simulink model "tensegrity_joint_universal"  (R2022b)
settings: Solver=VariableStepAuto  StartTime=0.0  StopTime=t_end  RelTol=1e-3
InitFcn:
  | %parameters_tensegrity_joint;
  | %l0_all=cables_l0(fix, fiz, w, h, b);
  | %predpeti=0.95;
values from neighbouring files (symbols this model uses):
  Fx_load = joint_stiffness(1, 12)    [plot_graphs_revolute.m]    (also in tensegrity_joint_revolute_stiffness.m = 10)
  Fy_load = joint_stiffness(1, 13)    [plot_graphs_revolute.m]    (also in tensegrity_joint_revolute_stiffness.m = 0)
  Fz_load = joint_stiffness(1, 14)    [plot_graphs_revolute.m]    (also in tensegrity_joint_revolute_stiffness.m = 0)
  l0_all = [l01, l02, l03, l04, l05, l06, l07, l08]    [tensegrity_universal_joint_plot.m]
  Mx_load = joint_stiffness(1, 15)    [plot_graphs_revolute.m]    (also in tensegrity_joint_revolute_stiffness.m = 0)
  My_load = joint_stiffness(1, 16)    [plot_graphs_revolute.m]    (also in tensegrity_joint_revolute_stiffness.m = 0)
  Mz_load = joint_stiffness(1, 17)    [plot_graphs_revolute.m]    (also in tensegrity_joint_revolute_stiffness.m = 0)
  predpeti_all = ll./l0_all    [tensegrity_joint_revolute_stiffness.m]
  t_measure = 0.25    [tensegrity_joint_revolute_stiffness.m]
undefined symbols (not defined in the file or in its folder): a, b, b_all, h, k_all, w
libraries: nesl_utility x35, sm_lib x33
(part 2 of 2)

== system tensegrity_joint_universal/Subsystem/internal cable force_3/cable force ==
  i : Inport
  PS-Simulink Converter1 : nesl_utility/PS-Simulink Converter  PhysicalDomain=network_engine_domain  SubClassName=ps_output  LeftPortType=input  RightPortType=output  PseudoPeriodic=off  Frequencies=[]  VectorFormat=1-D array  Unit=inherit  AffineConversion=off
  PS-Simulink Converter2 : nesl_utility/PS-Simulink Converter  PhysicalDomain=network_engine_domain  SubClassName=ps_output  LeftPortType=input  RightPortType=output  PseudoPeriodic=off  Frequencies=[]  VectorFormat=1-D array  Unit=inherit  AffineConversion=off
  Transform Sensor : sm_lib/Frames and Transforms/Transform Sensor  MeasurementFrame=World  SenseAngle=off  SenseAxis=off  SenseQ=off  SenseR=off  SenseRotationSequence=off  RotationSequence=XYX  SenseOmegaX=off  SenseOmegaY=off  SenseOmegaZ=off  SenseQDot=off  SenseRDot=off  SenseAlphaX=off  SenseAlphaY=off  SenseAlphaZ=off  SenseQDDot=off  SenseRDDot=off  SenseX=off  SenseY=off  SenseZ=off  SenseRad=off  SenseAzim=off  SenseDist=on  SenseInc=off  SenseXDot=off  SenseYDot=off  SenseZDot=off  SenseRadDot=off  SenseAzimDot=off  SenseDistDot=on  SenseIncDot=off  SenseXDDot=off  SenseYDDot=off  SenseZDDot=off  SenseRadDDot=off  SenseAzimDDot=off  SenseDistDDot=off  SenseIncDDot=off
  cable force computation : MATLAB Function  TreatAsAtomicUnit=on
  parameter selection : Subsystem
  TO : PMIOPort  Side=Right
  FROM : PMIOPort  Port=2  Side=Right
  Fc : Outport
  wires:
  cable force computation/1(Fc) -> Fc/1
  parameter selection/2(b) -> cable force computation/2(b)
  parameter selection/1(k) -> cable force computation/1(k)
  PS-Simulink Converter1/1 -> cable force computation/4(l)
  PS-Simulink Converter2/1 -> cable force computation/5(v)
  i/1 -> parameter selection/1(i)
  parameter selection/4(l0_p) -> cable force computation/3(l0)
  connections:
  Transform Sensor/RConn3 -- PS-Simulink Converter2/LConn1
  Transform Sensor/RConn2 -- PS-Simulink Converter1/LConn1
  Transform Sensor/RConn1 -- TO/RConn1
  Transform Sensor/LConn1 -- FROM/RConn1

== system tensegrity_joint_universal/Subsystem/internal cable force_4/cable force ==
  i : Inport
  PS-Simulink Converter1 : nesl_utility/PS-Simulink Converter  PhysicalDomain=network_engine_domain  SubClassName=ps_output  LeftPortType=input  RightPortType=output  PseudoPeriodic=off  Frequencies=[]  VectorFormat=1-D array  Unit=inherit  AffineConversion=off
  PS-Simulink Converter2 : nesl_utility/PS-Simulink Converter  PhysicalDomain=network_engine_domain  SubClassName=ps_output  LeftPortType=input  RightPortType=output  PseudoPeriodic=off  Frequencies=[]  VectorFormat=1-D array  Unit=inherit  AffineConversion=off
  Transform Sensor : sm_lib/Frames and Transforms/Transform Sensor  MeasurementFrame=World  SenseAngle=off  SenseAxis=off  SenseQ=off  SenseR=off  SenseRotationSequence=off  RotationSequence=XYX  SenseOmegaX=off  SenseOmegaY=off  SenseOmegaZ=off  SenseQDot=off  SenseRDot=off  SenseAlphaX=off  SenseAlphaY=off  SenseAlphaZ=off  SenseQDDot=off  SenseRDDot=off  SenseX=off  SenseY=off  SenseZ=off  SenseRad=off  SenseAzim=off  SenseDist=on  SenseInc=off  SenseXDot=off  SenseYDot=off  SenseZDot=off  SenseRadDot=off  SenseAzimDot=off  SenseDistDot=on  SenseIncDot=off  SenseXDDot=off  SenseYDDot=off  SenseZDDot=off  SenseRadDDot=off  SenseAzimDDot=off  SenseDistDDot=off  SenseIncDDot=off
  cable force computation : MATLAB Function  TreatAsAtomicUnit=on
  parameter selection : Subsystem
  TO : PMIOPort  Side=Right
  FROM : PMIOPort  Port=2  Side=Right
  Fc : Outport
  wires:
  cable force computation/1(Fc) -> Fc/1
  parameter selection/2(b) -> cable force computation/2(b)
  parameter selection/1(k) -> cable force computation/1(k)
  PS-Simulink Converter1/1 -> cable force computation/4(l)
  PS-Simulink Converter2/1 -> cable force computation/5(v)
  i/1 -> parameter selection/1(i)
  parameter selection/4(l0_p) -> cable force computation/3(l0)
  connections:
  Transform Sensor/RConn3 -- PS-Simulink Converter2/LConn1
  Transform Sensor/RConn2 -- PS-Simulink Converter1/LConn1
  Transform Sensor/RConn1 -- TO/RConn1
  Transform Sensor/LConn1 -- FROM/RConn1

== system tensegrity_joint_universal/Subsystem/internal cable force_5/cable force ==
  i : Inport
  PS-Simulink Converter1 : nesl_utility/PS-Simulink Converter  PhysicalDomain=network_engine_domain  SubClassName=ps_output  LeftPortType=input  RightPortType=output  PseudoPeriodic=off  Frequencies=[]  VectorFormat=1-D array  Unit=inherit  AffineConversion=off
  PS-Simulink Converter2 : nesl_utility/PS-Simulink Converter  PhysicalDomain=network_engine_domain  SubClassName=ps_output  LeftPortType=input  RightPortType=output  PseudoPeriodic=off  Frequencies=[]  VectorFormat=1-D array  Unit=inherit  AffineConversion=off
  Transform Sensor : sm_lib/Frames and Transforms/Transform Sensor  MeasurementFrame=World  SenseAngle=off  SenseAxis=off  SenseQ=off  SenseR=off  SenseRotationSequence=off  RotationSequence=XYX  SenseOmegaX=off  SenseOmegaY=off  SenseOmegaZ=off  SenseQDot=off  SenseRDot=off  SenseAlphaX=off  SenseAlphaY=off  SenseAlphaZ=off  SenseQDDot=off  SenseRDDot=off  SenseX=off  SenseY=off  SenseZ=off  SenseRad=off  SenseAzim=off  SenseDist=on  SenseInc=off  SenseXDot=off  SenseYDot=off  SenseZDot=off  SenseRadDot=off  SenseAzimDot=off  SenseDistDot=on  SenseIncDot=off  SenseXDDot=off  SenseYDDot=off  SenseZDDot=off  SenseRadDDot=off  SenseAzimDDot=off  SenseDistDDot=off  SenseIncDDot=off
  cable force computation : MATLAB Function  TreatAsAtomicUnit=on
  parameter selection : Subsystem
  TO : PMIOPort  Side=Right
  FROM : PMIOPort  Port=2  Side=Right
  Fc : Outport
  wires:
  cable force computation/1(Fc) -> Fc/1
  parameter selection/2(b) -> cable force computation/2(b)
  parameter selection/1(k) -> cable force computation/1(k)
  PS-Simulink Converter1/1 -> cable force computation/4(l)
  PS-Simulink Converter2/1 -> cable force computation/5(v)
  i/1 -> parameter selection/1(i)
  parameter selection/4(l0_p) -> cable force computation/3(l0)
  connections:
  Transform Sensor/RConn3 -- PS-Simulink Converter2/LConn1
  Transform Sensor/RConn2 -- PS-Simulink Converter1/LConn1
  Transform Sensor/RConn1 -- TO/RConn1
  Transform Sensor/LConn1 -- FROM/RConn1

== system tensegrity_joint_universal/Subsystem/internal cable force_6/cable force ==
  i : Inport
  PS-Simulink Converter1 : nesl_utility/PS-Simulink Converter  PhysicalDomain=network_engine_domain  SubClassName=ps_output  LeftPortType=input  RightPortType=output  PseudoPeriodic=off  Frequencies=[]  VectorFormat=1-D array  Unit=inherit  AffineConversion=off
  PS-Simulink Converter2 : nesl_utility/PS-Simulink Converter  PhysicalDomain=network_engine_domain  SubClassName=ps_output  LeftPortType=input  RightPortType=output  PseudoPeriodic=off  Frequencies=[]  VectorFormat=1-D array  Unit=inherit  AffineConversion=off
  Transform Sensor : sm_lib/Frames and Transforms/Transform Sensor  MeasurementFrame=World  SenseAngle=off  SenseAxis=off  SenseQ=off  SenseR=off  SenseRotationSequence=off  RotationSequence=XYX  SenseOmegaX=off  SenseOmegaY=off  SenseOmegaZ=off  SenseQDot=off  SenseRDot=off  SenseAlphaX=off  SenseAlphaY=off  SenseAlphaZ=off  SenseQDDot=off  SenseRDDot=off  SenseX=off  SenseY=off  SenseZ=off  SenseRad=off  SenseAzim=off  SenseDist=on  SenseInc=off  SenseXDot=off  SenseYDot=off  SenseZDot=off  SenseRadDot=off  SenseAzimDot=off  SenseDistDot=on  SenseIncDot=off  SenseXDDot=off  SenseYDDot=off  SenseZDDot=off  SenseRadDDot=off  SenseAzimDDot=off  SenseDistDDot=off  SenseIncDDot=off
  cable force computation : MATLAB Function  TreatAsAtomicUnit=on
  parameter selection : Subsystem
  TO : PMIOPort  Side=Right
  FROM : PMIOPort  Port=2  Side=Right
  Fc : Outport
  wires:
  cable force computation/1(Fc) -> Fc/1
  parameter selection/2(b) -> cable force computation/2(b)
  parameter selection/1(k) -> cable force computation/1(k)
  PS-Simulink Converter1/1 -> cable force computation/4(l)
  PS-Simulink Converter2/1 -> cable force computation/5(v)
  i/1 -> parameter selection/1(i)
  parameter selection/4(l0_p) -> cable force computation/3(l0)
  connections:
  Transform Sensor/RConn3 -- PS-Simulink Converter2/LConn1
  Transform Sensor/RConn2 -- PS-Simulink Converter1/LConn1
  Transform Sensor/RConn1 -- TO/RConn1
  Transform Sensor/LConn1 -- FROM/RConn1

== system tensegrity_joint_universal/Subsystem/internal cable force_7/cable force ==
  i : Inport
  PS-Simulink Converter1 : nesl_utility/PS-Simulink Converter  PhysicalDomain=network_engine_domain  SubClassName=ps_output  LeftPortType=input  RightPortType=output  PseudoPeriodic=off  Frequencies=[]  VectorFormat=1-D array  Unit=inherit  AffineConversion=off
  PS-Simulink Converter2 : nesl_utility/PS-Simulink Converter  PhysicalDomain=network_engine_domain  SubClassName=ps_output  LeftPortType=input  RightPortType=output  PseudoPeriodic=off  Frequencies=[]  VectorFormat=1-D array  Unit=inherit  AffineConversion=off
  Transform Sensor : sm_lib/Frames and Transforms/Transform Sensor  MeasurementFrame=World  SenseAngle=off  SenseAxis=off  SenseQ=off  SenseR=off  SenseRotationSequence=off  RotationSequence=XYX  SenseOmegaX=off  SenseOmegaY=off  SenseOmegaZ=off  SenseQDot=off  SenseRDot=off  SenseAlphaX=off  SenseAlphaY=off  SenseAlphaZ=off  SenseQDDot=off  SenseRDDot=off  SenseX=off  SenseY=off  SenseZ=off  SenseRad=off  SenseAzim=off  SenseDist=on  SenseInc=off  SenseXDot=off  SenseYDot=off  SenseZDot=off  SenseRadDot=off  SenseAzimDot=off  SenseDistDot=on  SenseIncDot=off  SenseXDDot=off  SenseYDDot=off  SenseZDDot=off  SenseRadDDot=off  SenseAzimDDot=off  SenseDistDDot=off  SenseIncDDot=off
  cable force computation : MATLAB Function  TreatAsAtomicUnit=on
  parameter selection : Subsystem
  TO : PMIOPort  Side=Right
  FROM : PMIOPort  Port=2  Side=Right
  Fc : Outport
  wires:
  cable force computation/1(Fc) -> Fc/1
  parameter selection/2(b) -> cable force computation/2(b)
  parameter selection/1(k) -> cable force computation/1(k)
  PS-Simulink Converter1/1 -> cable force computation/4(l)
  PS-Simulink Converter2/1 -> cable force computation/5(v)
  i/1 -> parameter selection/1(i)
  parameter selection/4(l0_p) -> cable force computation/3(l0)
  connections:
  Transform Sensor/RConn3 -- PS-Simulink Converter2/LConn1
  Transform Sensor/RConn2 -- PS-Simulink Converter1/LConn1
  Transform Sensor/RConn1 -- TO/RConn1
  Transform Sensor/LConn1 -- FROM/RConn1

== system tensegrity_joint_universal/Subsystem/internal cable force_8/cable force ==
  i : Inport
  PS-Simulink Converter1 : nesl_utility/PS-Simulink Converter  PhysicalDomain=network_engine_domain  SubClassName=ps_output  LeftPortType=input  RightPortType=output  PseudoPeriodic=off  Frequencies=[]  VectorFormat=1-D array  Unit=inherit  AffineConversion=off
  PS-Simulink Converter2 : nesl_utility/PS-Simulink Converter  PhysicalDomain=network_engine_domain  SubClassName=ps_output  LeftPortType=input  RightPortType=output  PseudoPeriodic=off  Frequencies=[]  VectorFormat=1-D array  Unit=inherit  AffineConversion=off
  Transform Sensor : sm_lib/Frames and Transforms/Transform Sensor  MeasurementFrame=World  SenseAngle=off  SenseAxis=off  SenseQ=off  SenseR=off  SenseRotationSequence=off  RotationSequence=XYX  SenseOmegaX=off  SenseOmegaY=off  SenseOmegaZ=off  SenseQDot=off  SenseRDot=off  SenseAlphaX=off  SenseAlphaY=off  SenseAlphaZ=off  SenseQDDot=off  SenseRDDot=off  SenseX=off  SenseY=off  SenseZ=off  SenseRad=off  SenseAzim=off  SenseDist=on  SenseInc=off  SenseXDot=off  SenseYDot=off  SenseZDot=off  SenseRadDot=off  SenseAzimDot=off  SenseDistDot=on  SenseIncDot=off  SenseXDDot=off  SenseYDDot=off  SenseZDDot=off  SenseRadDDot=off  SenseAzimDDot=off  SenseDistDDot=off  SenseIncDDot=off
  cable force computation : MATLAB Function  TreatAsAtomicUnit=on
  parameter selection : Subsystem
  TO : PMIOPort  Side=Right
  FROM : PMIOPort  Port=2  Side=Right
  Fc : Outport
  wires:
  cable force computation/1(Fc) -> Fc/1
  parameter selection/2(b) -> cable force computation/2(b)
  parameter selection/1(k) -> cable force computation/1(k)
  PS-Simulink Converter1/1 -> cable force computation/4(l)
  PS-Simulink Converter2/1 -> cable force computation/5(v)
  i/1 -> parameter selection/1(i)
  parameter selection/4(l0_p) -> cable force computation/3(l0)
  connections:
  Transform Sensor/RConn3 -- PS-Simulink Converter2/LConn1
  Transform Sensor/RConn2 -- PS-Simulink Converter1/LConn1
  Transform Sensor/RConn1 -- TO/RConn1
  Transform Sensor/LConn1 -- FROM/RConn1

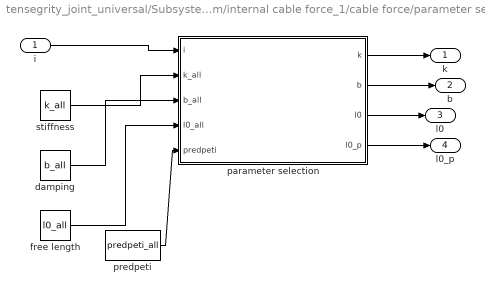
== system tensegrity_joint_universal/Subsystem/internal cable force_1/cable force/parameter selection ==
  i : Inport
  damping : Constant  Value=b_all
  free length : Constant  Value=l0_all
  parameter selection : MATLAB Function  TreatAsAtomicUnit=on
  predpeti : Constant  Value=predpeti_all
  stiffness : Constant  Value=k_all
  k : Outport
  b : Outport  Port=2
  l0 : Outport  Port=3
  l0_p : Outport  Port=4
  wires:
  damping/1 -> parameter selection/3(b_all)
  stiffness/1 -> parameter selection/2(k_all)
  free length/1 -> parameter selection/4(l0_all)
  parameter selection/2(b) -> b/1
  i/1 -> parameter selection/1(i)
  parameter selection/3(l0) -> l0/1
  parameter selection/1(k) -> k/1
  parameter selection/4(l0_p) -> l0_p/1
  predpeti/1 -> parameter selection/5(predpeti)

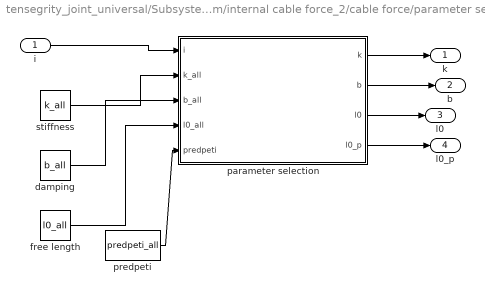
== system tensegrity_joint_universal/Subsystem/internal cable force_2/cable force/parameter selection ==
  i : Inport
  damping : Constant  Value=b_all
  free length : Constant  Value=l0_all
  parameter selection : MATLAB Function  TreatAsAtomicUnit=on
  predpeti : Constant  Value=predpeti_all
  stiffness : Constant  Value=k_all
  k : Outport
  b : Outport  Port=2
  l0 : Outport  Port=3
  l0_p : Outport  Port=4
  wires:
  damping/1 -> parameter selection/3(b_all)
  stiffness/1 -> parameter selection/2(k_all)
  free length/1 -> parameter selection/4(l0_all)
  parameter selection/2(b) -> b/1
  i/1 -> parameter selection/1(i)
  parameter selection/3(l0) -> l0/1
  parameter selection/1(k) -> k/1
  parameter selection/4(l0_p) -> l0_p/1
  predpeti/1 -> parameter selection/5(predpeti)

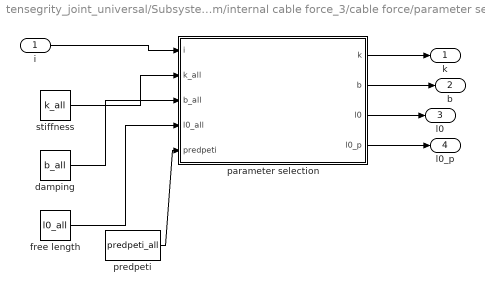
== system tensegrity_joint_universal/Subsystem/internal cable force_3/cable force/parameter selection ==
  i : Inport
  damping : Constant  Value=b_all
  free length : Constant  Value=l0_all
  parameter selection : MATLAB Function  TreatAsAtomicUnit=on
  predpeti : Constant  Value=predpeti_all
  stiffness : Constant  Value=k_all
  k : Outport
  b : Outport  Port=2
  l0 : Outport  Port=3
  l0_p : Outport  Port=4
  wires:
  damping/1 -> parameter selection/3(b_all)
  stiffness/1 -> parameter selection/2(k_all)
  free length/1 -> parameter selection/4(l0_all)
  parameter selection/2(b) -> b/1
  i/1 -> parameter selection/1(i)
  parameter selection/3(l0) -> l0/1
  parameter selection/1(k) -> k/1
  parameter selection/4(l0_p) -> l0_p/1
  predpeti/1 -> parameter selection/5(predpeti)

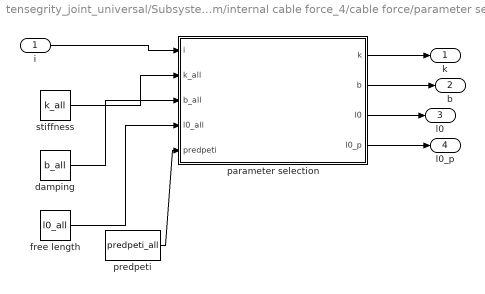
== system tensegrity_joint_universal/Subsystem/internal cable force_4/cable force/parameter selection ==
  i : Inport
  damping : Constant  Value=b_all
  free length : Constant  Value=l0_all
  parameter selection : MATLAB Function  TreatAsAtomicUnit=on
  predpeti : Constant  Value=predpeti_all
  stiffness : Constant  Value=k_all
  k : Outport
  b : Outport  Port=2
  l0 : Outport  Port=3
  l0_p : Outport  Port=4
  wires:
  damping/1 -> parameter selection/3(b_all)
  stiffness/1 -> parameter selection/2(k_all)
  free length/1 -> parameter selection/4(l0_all)
  parameter selection/2(b) -> b/1
  i/1 -> parameter selection/1(i)
  parameter selection/3(l0) -> l0/1
  parameter selection/1(k) -> k/1
  parameter selection/4(l0_p) -> l0_p/1
  predpeti/1 -> parameter selection/5(predpeti)

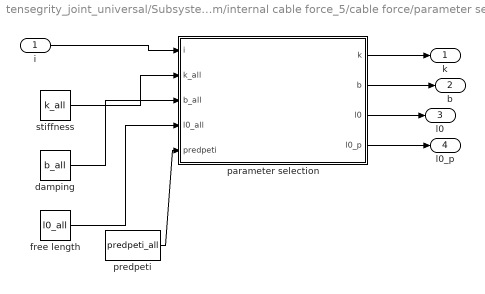
== system tensegrity_joint_universal/Subsystem/internal cable force_5/cable force/parameter selection ==
  i : Inport
  damping : Constant  Value=b_all
  free length : Constant  Value=l0_all
  parameter selection : MATLAB Function  TreatAsAtomicUnit=on
  predpeti : Constant  Value=predpeti_all
  stiffness : Constant  Value=k_all
  k : Outport
  b : Outport  Port=2
  l0 : Outport  Port=3
  l0_p : Outport  Port=4
  wires:
  damping/1 -> parameter selection/3(b_all)
  stiffness/1 -> parameter selection/2(k_all)
  free length/1 -> parameter selection/4(l0_all)
  parameter selection/2(b) -> b/1
  i/1 -> parameter selection/1(i)
  parameter selection/3(l0) -> l0/1
  parameter selection/1(k) -> k/1
  parameter selection/4(l0_p) -> l0_p/1
  predpeti/1 -> parameter selection/5(predpeti)

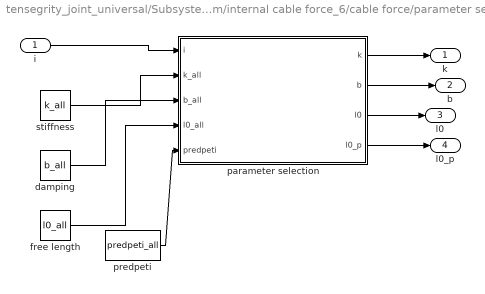
== system tensegrity_joint_universal/Subsystem/internal cable force_6/cable force/parameter selection ==
  i : Inport
  damping : Constant  Value=b_all
  free length : Constant  Value=l0_all
  parameter selection : MATLAB Function  TreatAsAtomicUnit=on
  predpeti : Constant  Value=predpeti_all
  stiffness : Constant  Value=k_all
  k : Outport
  b : Outport  Port=2
  l0 : Outport  Port=3
  l0_p : Outport  Port=4
  wires:
  damping/1 -> parameter selection/3(b_all)
  stiffness/1 -> parameter selection/2(k_all)
  free length/1 -> parameter selection/4(l0_all)
  parameter selection/2(b) -> b/1
  i/1 -> parameter selection/1(i)
  parameter selection/3(l0) -> l0/1
  parameter selection/1(k) -> k/1
  parameter selection/4(l0_p) -> l0_p/1
  predpeti/1 -> parameter selection/5(predpeti)

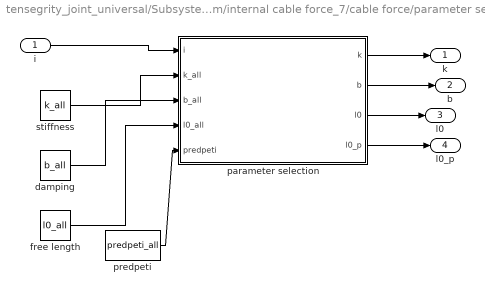
== system tensegrity_joint_universal/Subsystem/internal cable force_7/cable force/parameter selection ==
  i : Inport
  damping : Constant  Value=b_all
  free length : Constant  Value=l0_all
  parameter selection : MATLAB Function  TreatAsAtomicUnit=on
  predpeti : Constant  Value=predpeti_all
  stiffness : Constant  Value=k_all
  k : Outport
  b : Outport  Port=2
  l0 : Outport  Port=3
  l0_p : Outport  Port=4
  wires:
  damping/1 -> parameter selection/3(b_all)
  stiffness/1 -> parameter selection/2(k_all)
  free length/1 -> parameter selection/4(l0_all)
  parameter selection/2(b) -> b/1
  i/1 -> parameter selection/1(i)
  parameter selection/3(l0) -> l0/1
  parameter selection/1(k) -> k/1
  parameter selection/4(l0_p) -> l0_p/1
  predpeti/1 -> parameter selection/5(predpeti)

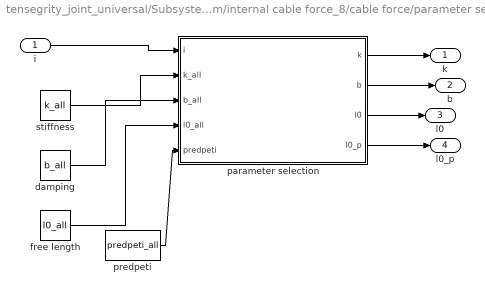
== system tensegrity_joint_universal/Subsystem/internal cable force_8/cable force/parameter selection ==
  i : Inport
  damping : Constant  Value=b_all
  free length : Constant  Value=l0_all
  parameter selection : MATLAB Function  TreatAsAtomicUnit=on
  predpeti : Constant  Value=predpeti_all
  stiffness : Constant  Value=k_all
  k : Outport
  b : Outport  Port=2
  l0 : Outport  Port=3
  l0_p : Outport  Port=4
  wires:
  damping/1 -> parameter selection/3(b_all)
  stiffness/1 -> parameter selection/2(k_all)
  free length/1 -> parameter selection/4(l0_all)
  parameter selection/2(b) -> b/1
  i/1 -> parameter selection/1(i)
  parameter selection/3(l0) -> l0/1
  parameter selection/1(k) -> k/1
  parameter selection/4(l0_p) -> l0_p/1
  predpeti/1 -> parameter selection/5(predpeti)

== matlab function tensegrity_joint_universal/Subsystem/internal cable force_5/cable force/parameter selection/parameter selection ==
  data: i input; k output; k_all input; b_all input; l0_all input; b output; l0 output; l0_p output; predpeti input
function [k, b, l0, l0_p] = parameter_selection(i, k_all, b_all, l0_all, predpeti)

k=k_all(i);
b=b_all(i);
l0=l0_all(i);
l0_p=l0_all(i)*predpeti(i);

== matlab function tensegrity_joint_universal/Subsystem/internal cable force_6/cable force/cable force computation ==
  data: k input; Fc output; b input; l0 input; l input; v input
function Fc = cable_force(k, b,l0, l, v)

Fc=k*(l-l0) + b*v;

== matlab function tensegrity_joint_universal/Subsystem/internal cable force_6/cable force/parameter selection/parameter selection ==
  data: i input; k output; k_all input; b_all input; l0_all input; b output; l0 output; l0_p output; predpeti input
function [k, b, l0, l0_p] = parameter_selection(i, k_all, b_all, l0_all, predpeti)

k=k_all(i);
b=b_all(i);
l0=l0_all(i);
l0_p=l0_all(i)*predpeti(i);

== matlab function tensegrity_joint_universal/Subsystem/internal cable force_7/cable force/cable force computation ==
  data: k input; Fc output; b input; l0 input; l input; v input
function Fc = cable_force(k, b,l0, l, v)

Fc=k*(l-l0) + b*v;

== matlab function tensegrity_joint_universal/Subsystem/internal cable force_2/cable force/cable force computation ==
  data: k input; Fc output; b input; l0 input; l input; v input
function Fc = cable_force(k, b,l0, l, v)

Fc=k*(l-l0) + b*v;

== matlab function tensegrity_joint_universal/Subsystem/internal cable force_7/cable force/parameter selection/parameter selection ==
  data: i input; k output; k_all input; b_all input; l0_all input; b output; l0 output; l0_p output; predpeti input
function [k, b, l0, l0_p] = parameter_selection(i, k_all, b_all, l0_all, predpeti)

k=k_all(i);
b=b_all(i);
l0=l0_all(i);
l0_p=l0_all(i)*predpeti(i);

== matlab function tensegrity_joint_universal/Subsystem/internal cable force_8/cable force/cable force computation ==
  data: k input; Fc output; b input; l0 input; l input; v input
function Fc = cable_force(k, b,l0, l, v)

Fc=k*(l-l0) + b*v;

== matlab function tensegrity_joint_universal/Subsystem/internal cable force_8/cable force/parameter selection/parameter selection ==
  data: i input; k output; k_all input; b_all input; l0_all input; b output; l0 output; l0_p output; predpeti input
function [k, b, l0, l0_p] = parameter_selection(i, k_all, b_all, l0_all, predpeti)

k=k_all(i);
b=b_all(i);
l0=l0_all(i);
l0_p=l0_all(i)*predpeti(i);

== matlab function tensegrity_joint_universal/Subsystem/internal cable force_1/cable force/cable force computation ==
  data: k input; Fc output; b input; l0 input; l input; v input
function Fc = cable_force(k, b,l0, l, v)

Fc=k*(l-l0) + b*v;

== matlab function tensegrity_joint_universal/Subsystem/internal cable force_1/cable force/parameter selection/parameter selection ==
  data: i input; k output; k_all input; b_all input; l0_all input; b output; l0 output; l0_p output; predpeti input
function [k, b, l0, l0_p] = parameter_selection(i, k_all, b_all, l0_all, predpeti)

k=k_all(i);
b=b_all(i);
l0=l0_all(i);
l0_p=l0_all(i)*predpeti(i);

== matlab function tensegrity_joint_universal/Subsystem/internal cable force_2/cable force/parameter selection/parameter selection ==
  data: i input; k output; k_all input; b_all input; l0_all input; b output; l0 output; l0_p output; predpeti input
function [k, b, l0, l0_p] = parameter_selection(i, k_all, b_all, l0_all, predpeti)

k=k_all(i);
b=b_all(i);
l0=l0_all(i);
l0_p=l0_all(i)*predpeti(i);

== matlab function tensegrity_joint_universal/Subsystem/internal cable force_3/cable force/cable force computation ==
  data: k input; Fc output; b input; l0 input; l input; v input
function Fc = cable_force(k, b,l0, l, v)

Fc=k*(l-l0) + b*v;

== matlab function tensegrity_joint_universal/Subsystem/internal cable force_3/cable force/parameter selection/parameter selection ==
  data: i input; k output; k_all input; b_all input; l0_all input; b output; l0 output; l0_p output; predpeti input
function [k, b, l0, l0_p] = parameter_selection(i, k_all, b_all, l0_all, predpeti)

k=k_all(i);
b=b_all(i);
l0=l0_all(i);
l0_p=l0_all(i)*predpeti(i);

== matlab function tensegrity_joint_universal/Subsystem/internal cable force_4/cable force/cable force computation ==
  data: k input; Fc output; b input; l0 input; l input; v input
function Fc = cable_force(k, b,l0, l, v)

Fc=k*(l-l0) + b*v;

== matlab function tensegrity_joint_universal/Subsystem/internal cable force_4/cable force/parameter selection/parameter selection ==
  data: i input; k output; k_all input; b_all input; l0_all input; b output; l0 output; l0_p output; predpeti input
function [k, b, l0, l0_p] = parameter_selection(i, k_all, b_all, l0_all, predpeti)

k=k_all(i);
b=b_all(i);
l0=l0_all(i);
l0_p=l0_all(i)*predpeti(i);

== matlab function tensegrity_joint_universal/Subsystem/internal cable force_5/cable force/cable force computation ==
  data: k input; Fc output; b input; l0 input; l input; v input
function Fc = cable_force(k, b,l0, l, v)

Fc=k*(l-l0) + b*v;
